simulink model "followline"  (R2021b)
settings: Solver=FixedStepAuto  StartTime=0.0  StopTime=2  FixedStep=1e-3  RelTol=1e-3
values from neighbouring files (symbols this model uses):
  xr = -1    [avaliarFollowline.m]
  y0 = y0s(i)    [avaliarLinearidadeLateral.m]
  yr = yrs(j)    [avaliarFollowline.m]
undefined symbols (not defined in the file or in its folder): Kpsi, Kx, KyPrime, l, maxWheelSpeed, psi0, psirMax, r, vMax, vMin, x0
settings Model: Creator=mmaximo  LastModifiedBy=buga
settings SolverCC: AlgebraicLoopSolver=TrustRegion
settings DebuggingCC: SFMachineParentedDataDiag=warning

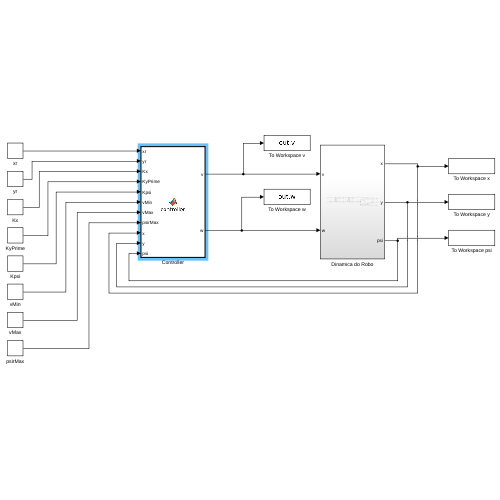
[thumbnail: Simulink's stored preview of the top-level diagram]
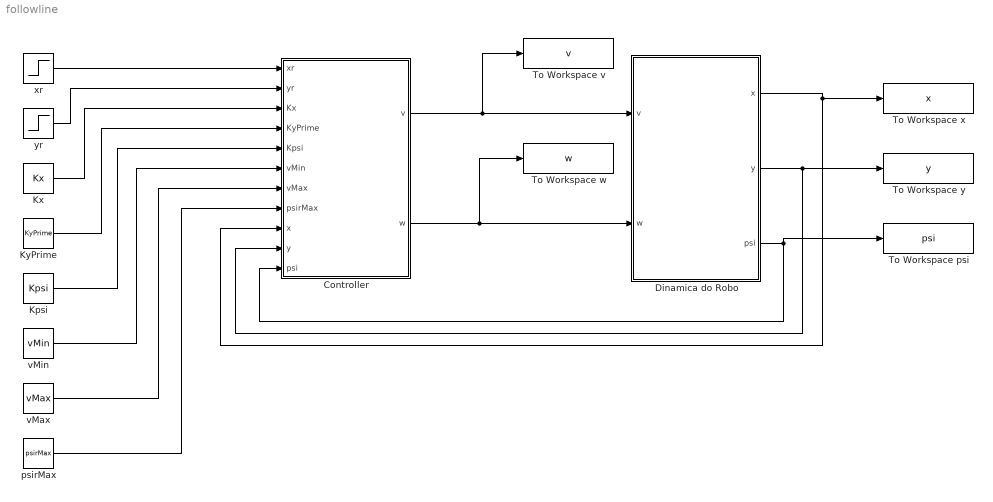
== system followline ==
  Controller : MATLAB Function  TreatAsAtomicUnit=on
  Dinamica do Robo : Subsystem
  Kpsi : Constant  Value=Kpsi
  Kx : Constant  Value=Kx
  KyPrime : Constant  Value=KyPrime
  To Workspace psi : ToWorkspace  VariableName=psi  SaveFormat=Structure With Time  SampleTime=-1
  To Workspace v : ToWorkspace  VariableName=v  SaveFormat=Structure With Time  SampleTime=-1
  To Workspace w : ToWorkspace  VariableName=w  SaveFormat=Structure With Time  SampleTime=-1
  To Workspace x : ToWorkspace  VariableName=x  SaveFormat=Structure With Time  SampleTime=-1
  To Workspace y : ToWorkspace  VariableName=y  SaveFormat=Structure With Time  SampleTime=-1
  psirMax : Constant  Value=psirMax
  vMax : Constant  Value=vMax
  vMin : Constant  Value=vMin
  xr : Step  Time=0  After=xr  SampleTime=0
  yr : Step  Time=0  After=yr  SampleTime=0
  wires:
  Controller/1(v) -> To Workspace v/1, Dinamica do Robo/1(v)
  Controller/2(w) -> To Workspace w/1, Dinamica do Robo/2(w)
  Kx/1 -> Controller/3(Kx)
  KyPrime/1 -> Controller/4(KyPrime)
  Kpsi/1 -> Controller/5(Kpsi)
  vMin/1 -> Controller/6(vMin)
  xr/1 -> Controller/1(xr)
  yr/1 -> Controller/2(yr)
  Dinamica do Robo/1(x) -> Controller/9(x), To Workspace x/1
  Dinamica do Robo/2(y) -> Controller/10(y), To Workspace y/1
  Dinamica do Robo/3(psi) -> To Workspace psi/1, Controller/11(psi)
  psirMax/1 -> Controller/8(psirMax)
  vMax/1 -> Controller/7(vMax)

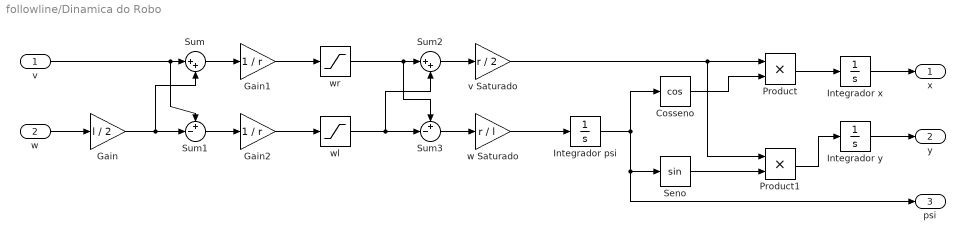
== system followline/Dinamica do Robo ==
  v : Inport
  w : Inport  Port=2
  Cosseno : Trigonometry  Operator=cos
  Gain : Gain  Gain=l / 2
  Gain1 : Gain  Gain=1 / r
  Gain2 : Gain  Gain=1 / r
  Integrador psi : Integrator  InitialCondition=psi0
  Integrador x : Integrator  InitialCondition=x0
  Integrador y : Integrator  InitialCondition=y0
  Product : Product
  Product1 : Product
  Seno : Trigonometry
  Sum : Sum  Inputs=|++
  Sum1 : Sum  Inputs=+-|
  Sum2 : Sum  Inputs=|++
  Sum3 : Sum  Inputs=+-|
  v Saturado : Gain  Gain=r / 2
  w Saturado : Gain  Gain=r / l
  wl : Saturate  UpperLimit=maxWheelSpeed  LowerLimit=-maxWheelSpeed
  wr : Saturate  UpperLimit=maxWheelSpeed  LowerLimit=-maxWheelSpeed
  x : Outport
  y : Outport  Port=2
  psi : Outport  Port=3
  wires:
  Integrador psi/1 -> Seno/1, psi/1, Cosseno/1
  Cosseno/1 -> Product/2
  Seno/1 -> Product1/2
  Product1/1 -> Integrador y/1
  Integrador y/1 -> y/1
  Product/1 -> Integrador x/1
  Integrador x/1 -> x/1
  w/1 -> Gain/1
  v/1 -> Sum1/1, Sum/1
  Gain/1 -> Sum1/2, Sum/2
  Sum1/1 -> Gain2/1
  Sum/1 -> Gain1/1
  Gain1/1 -> wr/1
  Gain2/1 -> wl/1
  wr/1 -> Sum3/1, Sum2/1
  wl/1 -> Sum3/2, Sum2/2
  Sum2/1 -> v Saturado/1
  Sum3/1 -> w Saturado/1
  w Saturado/1 -> Integrador psi/1
  v Saturado/1 -> Product1/1, Product/1

== matlab function followline/Controller ==
  data: v output; w output; xr input; yr input; Kx input; KyPrime input; Kpsi input; vMin input; vMax input; psirMax input; x input; y input; psi input
function [v, w] = controller(xr, yr, Kx, KyPrime, Kpsi, vMin, vMax, psirMax, x, y, psi)
% Implementa um controlador para um robo seguir uma linha, parando em um 
% ponto dessa linha.
% xr: referencia de x (ponto na linha).
% yr: referencia de posicao da linha.
% Kx: ganho proporcional do controlador frontal.
% KyPrime: parte constante do ganho de posicao do controlador lateral
% Kpsi: ganho de velocidade (angulo) do controlador lateral.
% vMin: velocidade minima usada na adaptacao de Ky.
% vMax: velocidade maxima comandada para o robo.
% psirMax: referencia de angulo maxima (saturacao).
% x: coordenada x da posicao atual do robo.
% y: coordenada y da posicao atual do robo.
% psi: orientacao atual.

% Implementar controlador completo
v = Kx*(xr -x);
v = min(vMax, max(-vMax, v));
if abs(v) > vMin
    Ky = KyPrime/v;
else
    Ky = KyPrime/vMin * sign(v);
end
psir = Ky*(yr - y);
psir = min(psirMax, max(-psirMax, psir));

w = Kpsi*(psir - psi);
end
